simulink library "calc_pqrHat_ul"  (R2020a)
settings: Solver=VariableStepAuto  StartTime=0.0  StopTime=10.0  RelTol=1e-3
values from neighbouring files (symbols this model uses):
  refChord = 0.55    [calcAeroCoefficients_ts.m]
  refSpan = 5.5    [calcAeroCoefficients_ts.m]
settings Model: Creator=Ayaz  LastModifiedBy=Ayaz

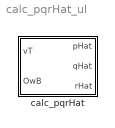
== system calc_pqrHat_ul ==
  calc_pqrHat : Subsystem  mask{refSpan=refSpan, refChord=refChord}
      mask prompts: refSpan "Reference wing span [m]"; refChord "Reference wing chord [m]"
      mask TypeOptions refSpan: Constant/Value
      mask TypeOptions refChord: Constant1/Value

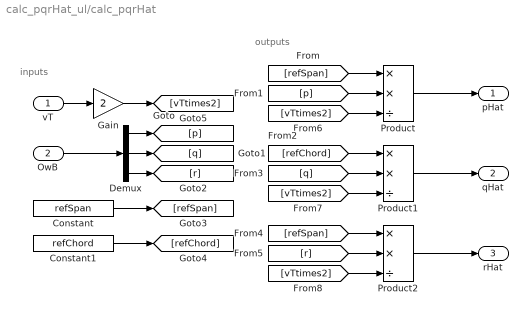
== system calc_pqrHat_ul/calc_pqrHat ==
  note: outputs
  note: inputs
  vT : Inport
  OwB : Inport  Port=2
  Constant : Constant  Value=refSpan
  Constant1 : Constant  Value=refChord
  Demux : Demux  Outputs=3
  Gain : Gain  Gain=2
  Product : Product  Inputs=**/
  Product1 : Product  Inputs=**/
  Product2 : Product  Inputs=**/
  pHat : Outport
  qHat : Outport  Port=2
  rHat : Outport  Port=3
  wires:
  OwB/1 -> Demux/1
  Demux/1 -> [p]
  Demux/2 -> [q]
  Demux/3 -> [r]
  Constant/1 -> [refSpan]
  Constant1/1 -> [refChord]
  vT/1 -> Gain/1
  [refSpan] -> Product/1
  [p] -> Product/2
  [vTtimes2] -> Product/3
  [refChord] -> Product1/1
  [q] -> Product1/2
  [vTtimes2] -> Product1/3
  [refSpan] -> Product2/1
  [r] -> Product2/2
  [vTtimes2] -> Product2/3
  Gain/1 -> [vTtimes2]
  Product/1 -> pHat/1
  Product1/1 -> qHat/1
  Product2/1 -> rHat/1
